simulink model "HeartBeat_Xor"  (R2014a)
settings: Solver=VariableStepAuto  StartTime=0.0  StopTime=100.0  RelTol=1e-3
libraries: commutil2 x2, simulink x1, simulink_extras x1
settings Model: Creator=RamPrasadh  LastModifiedBy=narayan
settings DataIOCC: SaveFormat=Dataset
settings OptimizationCC: SimCompilerOptimization=off
settings DebuggingCC: MergeDetectMultiDrivingBlocksExec=error  SolverPrmCheckMsg=none  FrameProcessingCompatibilityMsg=error  AllowSymbolicDim=off
settings HardwareCC: ProdBitPerPointer=64  ProdLargestAtomicFloat=Float  ProdIntDivRoundTo=Zero  ProdEndianess=LittleEndian  ProdWordSize=64  ProdHWDeviceType=Intel->x86-64 (Windows64)
settings RTWCC: RTWCompilerOptimization=off
settings GRTTargetCC: GeneratePreprocessorConditionals=Use local settings
settings ConfigComp: CovMetricSettings=dw  CovHtmlReporting=on  CovSaveCumulativeToWorkspaceVar=on  CovSaveSingleToWorkspaceVar=on  CovExternalEMLEnable=off

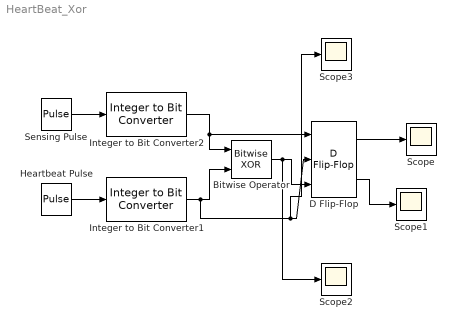
== system HeartBeat_Xor ==
  Bitwise Operator : simulink/Logic and Bit Operations/Bitwise Operator  logicop=XOR  UseBitMask=off  NumInputPorts=2  BitMask=bin2dec('11011001')  BitMaskRealWorld=Stored Integer
  D Flip-Flop : simulink_extras/Flip Flops/D Flip-Flop
  "Heartbeat Pulse " : DiscretePulseGenerator  Period=10  PulseWidth=5  PhaseDelay=1
  Integer to Bit Converter1 : commutil2/Integer to Bit Converter  nbits=3  signedInputValues=Unsigned  bitOrder=MSB first  outDtype=boolean
  Integer to Bit Converter2 : commutil2/Integer to Bit Converter  nbits=3  signedInputValues=Unsigned  bitOrder=MSB first  outDtype=boolean
  Scope{,1..3} (4 alike) : Scope
      Scope2 settings: SaveName=ScopeData2
      Scope3 settings: SaveName=ScopeData3
  "Sensing Pulse " : DiscretePulseGenerator  Period=10  PulseWidth=7
  wires:
  "Heartbeat Pulse "/1 -> Integer to Bit Converter1/1
  "Sensing Pulse "/1 -> Integer to Bit Converter2/1
  Integer to Bit Converter2/1 -> D Flip-Flop/1, Bitwise Operator/1
  Integer to Bit Converter1/1 -> Scope3/1, D Flip-Flop/2, Bitwise Operator/2
  D Flip-Flop/1 -> Scope/1
  D Flip-Flop/2 -> Scope1/1
  Bitwise Operator/1 -> Scope2/1, D Flip-Flop/3
